simulink model "RL_SAC"  (R2025a)
settings: Solver=FixedStepDiscrete  StartTime=0.0  StopTime=20  FixedStep=1e-2  RelTol=1e-6
undefined symbols (not defined in the file or in its folder): DiscIntNeverNeededParam
libraries: simulink x26, cstblocks x16, slpidlib x2, aerolibutil x2, rllib x1
(part 1 of 2)
settings Model: Creator=Rewse  LastModifiedBy=Rewse
settings SolverCC: ZeroCrossAlgorithm=Adaptive
settings DebuggingCC: IgnoredZcDiagnostic=none

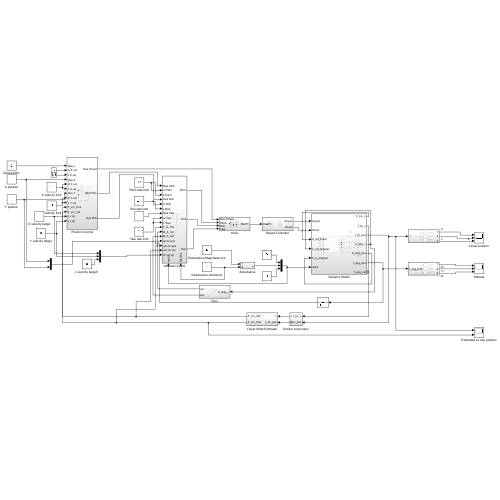
[thumbnail: Simulink's stored preview of the top-level diagram]
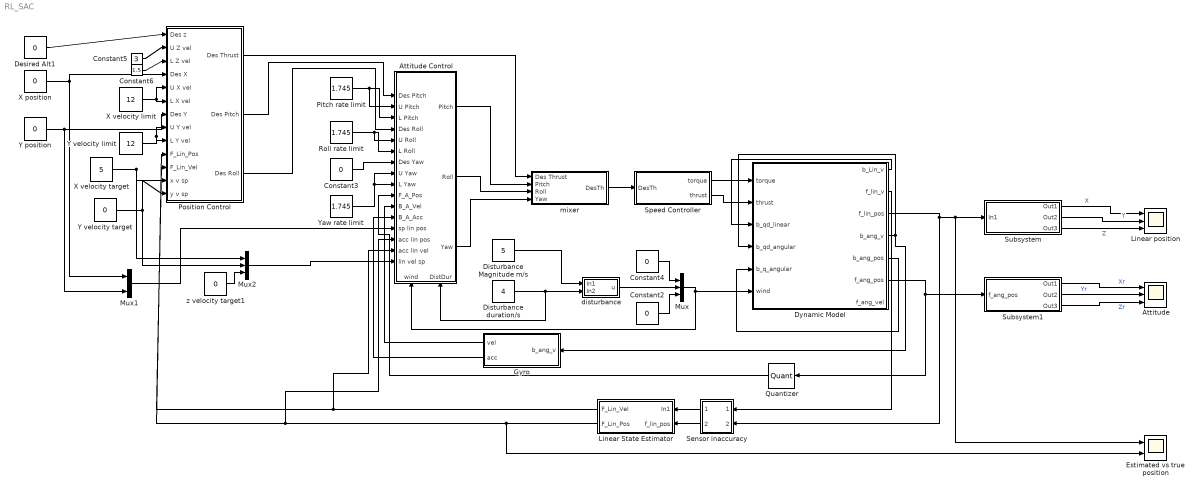
== system RL_SAC ==
  Attitude : Scope  NumInputPorts=3
      settings: ActiveDisplayYMinimum=-0.14361706032504082  ActiveDisplayYMaximum=0.032180546119047609
  Attitude Control : Subsystem
      settings: PortSchema="{\"entries\":[{\"content\":{\"sides\":[{\"content\":{\"connectorIds\":[\"In1\",\"In2\",\"In3\",\"In4\",\"In5\",\"In6\",\"In7\",\"In8\",\"In9\",\"In10\",\"In11\",\"In12\",\"In13\",\"In14\",\"In15\",\"In16\"]},\"type\":\"ConnectorPlacement.EquallySpacedRectSide\",\"uuid\":\"5aea7e22-cf15-44ef-b205-b6ced6f298a4\"},{\"content\":{\"connectorIds\":[\"Out1\",\"Out2\",\"Out3\"],\"side\":\"RIGHT\"},\"type\":\"ConnectorPlacement.EquallySpacedRectSide\",\"uuid\":\"9ef0269e-c37e-412a-be4f-a3e367ef4d40\"},{\"content\":{\"side\":\"TOP\"},\"type\":\"ConnectorPlacement.EquallySpacedRectSide\",\"uuid\":\"5b75e127-dd51-46ce-894a-a13043237b79\"},{\"content\":{\"connectorIds\":[\"In17\",\"In18\"],\"side\":\"BOTTOM\"},\"type\":\"ConnectorPlacement.EquallySpacedRectSide\",\"uuid\":\"a8713bdf-8295-4b8e-972b-b20a63c171f4\"}]},\"type\":\"ConnectorPlacement.EquallySpacedConnector\",\"uuid\":\"ff6dc2c6-b6a3-43bc-805b-8e42f8232d67\"}],\"packageUris\":[\"http://schema.mathworks.com/mf0/Connector/R2020b\"],\"version\":\"1.0\"}"
  Constant2 : Constant  Value=0
  Constant3 : Constant  Value=0
  Constant4 : Constant  Value=0
  Constant5 : Constant  Value=3
  Constant6 : Constant  Value=1.5
  Desired Alt1 : Constant  Value=0
  Disturbance Magnitude m/s : Constant  Value=5
  Disturbance duration/s : Constant  Value=4
  Dynamic Model : Subsystem
  Estimated vs true position : Scope  NumInputPorts=2
      settings: ActiveDisplayYMinimum=-18.877528524364443  ActiveDisplayYMaximum=162.40656098897554  DataLoggingVariableName=ScopeData4
  Gyro : Subsystem
  Linear State Estimator : Subsystem
  Linear position : Scope  NumInputPorts=3
      settings: ActiveDisplayYMinimum=-25.0677489650157  ActiveDisplayYMaximum=225.60952843294078
  Mux : Mux  Inputs=3
  Mux1 : Mux  Inputs=2
  Mux2 : Mux  Inputs=3
  Pitch rate limit : Constant  Value=1.745
  Position Control : Subsystem
  Quantizer : Quantizer  QuantizationInterval=0.01
  Roll rate limit : Constant  Value=1.745
  Sensor inaccuracy : Subsystem
  Speed Controller : Subsystem
  Subsystem : Subsystem
  Subsystem1 : Subsystem
  X position : Constant  Value=0
  X velocity limit : Constant  Value=12
  X velocity target : Constant  Value=5
  Y position : Constant  Value=0
  Y velocity limit : Constant  Value=12
  Y velocity target : Constant  Value=0
  Yaw rate limit : Constant  Value=1.745
  disturbance : Subsystem
  mixer : Subsystem
  z velocity target1 : Constant  Value=0
  wires:
  Subsystem/1(Out1) -> Linear position/1  "X"
  Subsystem/2(Out2) -> Linear position/2  "Y"
  Subsystem/3(Out3) -> Linear position/3  "Z"
  Subsystem1/1(Out1) -> Attitude/1  "Xr"
  Subsystem1/2(Out2) -> Attitude/2  "Yr"
  Subsystem1/3(Out3) -> Attitude/3  "Zr"
  Dynamic Model/5(b_ang_pos) -> Dynamic Model/5(b_q_angular)
  Dynamic Model/1(b_Lin_v) -> Dynamic Model/3(b_qd_linear)
  mixer/1(DesTh) -> Speed Controller/1(DesTh)
  Dynamic Model/4(b_ang_v) -> Gyro/1(b_ang_v), Dynamic Model/4(b_qd_angular)
  Attitude Control/1(Pitch) -> mixer/2(Pitch)
  Attitude Control/2(Roll) -> mixer/3(Roll)
  Pitch rate limit/1 -> Attitude Control/3(L Pitch), Attitude Control/2(U Pitch)
  Roll rate limit/1 -> Attitude Control/6(L Roll), Attitude Control/5(U Roll)
  Yaw rate limit/1 -> Attitude Control/8(U Yaw), Attitude Control/9(L Yaw)
  Constant3/1 -> Attitude Control/7(Des Yaw)
  Speed Controller/2(thrust) -> Dynamic Model/2(thrust)
  Speed Controller/1(torque) -> Dynamic Model/1(torque)
  Constant5/1 -> Position Control/2(U Z vel)
  Desired Alt1/1 -> Position Control/1(Des z)
  X velocity limit/1 -> Position Control/6(L X vel), Position Control/5(U X vel)
  Y velocity limit/1 -> Position Control/9(L Y vel), Position Control/8(U Y vel)
  Position Control/1(Des Thrust) -> mixer/1(Des Thrust)
  Constant6/1 -> Position Control/3(L Z vel)
  Y position/1 -> Mux1/2, Position Control/7(Des Y)
  Attitude Control/3(Yaw) -> mixer/4(Yaw)
  Gyro/1(vel) -> Attitude Control/11(B_A_Vel)
  Gyro/2(acc) -> Attitude Control/12(B_A_Acc)
  Dynamic Model/6(f_ang_pos) -> Quantizer/1, Subsystem1/1(f_ang_pos)
  X position/1 -> Mux1/1, Position Control/4(Des X)
  Constant2/1 -> Mux/3
  Sensor inaccuracy/2(Out2) -> Linear State Estimator/2(f_lin_pos)
  Sensor inaccuracy/1(Out1) -> Linear State Estimator/1(In1)
  Dynamic Model/2(f_lin_v) -> Sensor inaccuracy/1(f_lin_v)
  Dynamic Model/3(f_lin_pos) -> Sensor inaccuracy/2(f_lin_pos), Estimated vs true position/1, Subsystem/1(In1)
  Position Control/3(Des Roll) -> Attitude Control/4(Des Roll)
  Position Control/2(Des Pitch) -> Attitude Control/1(Des Pitch)
  Linear State Estimator/1(F_Lin_Vel) -> Attitude Control/15(acc lin vel), Position Control/11(F_Lin_Vel)
  Linear State Estimator/2(F_Lin_Pos) -> Estimated vs true position/2, Position Control/10(F_Lin_Pos), Attitude Control/14(acc lin pos)
  Mux1/1 -> Attitude Control/13(sp lin pos)
  Mux/1 -> Dynamic Model/6(wind), Attitude Control/17(wind)
  X velocity target/1 -> Mux2/1, Position Control/12(x v sp)
  Y velocity target/1 -> Mux2/2, Position Control/13(y v sp)
  Constant4/1 -> Mux/1
  Mux2/1 -> Attitude Control/16(lin vel sp)
  z velocity target1/1 -> Mux2/3
  Disturbance Magnitude m/s/1 -> disturbance/1(In1)
  disturbance/1(u) -> Mux/2
  Quantizer/1 -> Attitude Control/10(F_A_Pos)
  Disturbance duration/s/1 -> disturbance/2(In2), Attitude Control/18(DistDur)

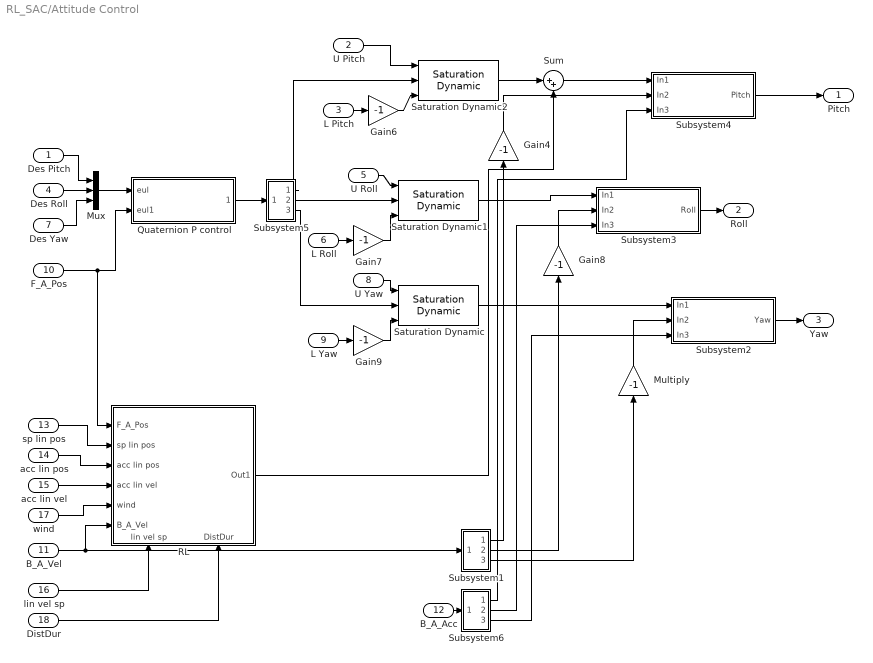
== system RL_SAC/Attitude Control ==
  Des Pitch : Inport
  U Pitch : Inport  Port=2
  L Pitch : Inport  Port=3
  Des Roll : Inport  Port=4
  U Roll : Inport  Port=5
  L Roll : Inport  Port=6
  Des Yaw : Inport  Port=7
  U Yaw : Inport  Port=8
  L Yaw : Inport  Port=9
  F_A_Pos : Inport  Port=10
  B_A_Vel : Inport  Port=11
  B_A_Acc : Inport  Port=12
  sp lin pos : Inport  Port=13
  acc lin pos : Inport  Port=14
  acc lin vel : Inport  Port=15
  lin vel sp : Inport  Port=16
  wind : Inport  Port=17
  DistDur : Inport  Port=18
  Gain{4,6..9} (5 alike) : Gain  Gain=-1
  Multiply : Gain  Gain=-1
  Mux : Mux  Inputs=3
  Quaternion P control : Subsystem
  RL : Subsystem
      settings: PortSchema="{\"entries\":[{\"content\":{\"sides\":[{\"content\":{\"connectorIds\":[\"In1\",\"In2\",\"In3\",\"In4\",\"In5\",\"In6\"]},\"type\":\"ConnectorPlacement.EquallySpacedRectSide\",\"uuid\":\"de9c2034-cd13-466b-8304-909c4731cac8\"},{\"content\":{\"connectorIds\":[\"Out1\"],\"side\":\"RIGHT\"},\"type\":\"ConnectorPlacement.EquallySpacedRectSide\",\"uuid\":\"4bbf1dae-6c36-474f-8444-ba23edf5e83e\"},{\"content\":{\"side\":\"TOP\"},\"type\":\"ConnectorPlacement.EquallySpacedRectSide\",\"uuid\":\"e128e6e1-e112-4b3d-a554-370c1b41a3dc\"},{\"content\":{\"connectorIds\":[\"In7\",\"In8\"],\"side\":\"BOTTOM\"},\"type\":\"ConnectorPlacement.EquallySpacedRectSide\",\"uuid\":\"ffd3f57f-9382-4033-b19c-cb1eae5b476f\"}]},\"type\":\"ConnectorPlacement.EquallySpacedConnector\",\"uuid\":\"d8782a20-2727-49b0-a468-40b427850214\"}],\"packageUris\":[\"http://schema.mathworks.com/mf0/Connector/R2020b\"],\"version\":\"1.0\"}"
  Saturation Dynamic : simulink/Discontinuities/Saturation Dynamic  OutMin=[]  OutMax=[]  OutDataTypeStr=Inherit: Same as second input  OutDataType=fixdt(1, 16)  OutScaling=2^-10  DoSatur=off
  Saturation Dynamic1 : simulink/Discontinuities/Saturation Dynamic  OutMin=[]  OutMax=[]  OutDataTypeStr=Inherit: Same as second input  OutDataType=fixdt(1, 16)  OutScaling=2^-10  DoSatur=off
  Saturation Dynamic2 : simulink/Discontinuities/Saturation Dynamic  OutMin=[]  OutMax=[]  OutDataTypeStr=Inherit: Same as second input  OutDataType=fixdt(1, 16)  OutScaling=2^-10  DoSatur=off
  Subsystem1 : Subsystem
  Subsystem2 : Subsystem
  Subsystem3 : Subsystem
  Subsystem4 : Subsystem
  Subsystem5 : Subsystem
  Subsystem6 : Subsystem
  Sum : Sum  Inputs=|++
  Pitch : Outport
  Roll : Outport  Port=2
  Yaw : Outport  Port=3
  wires:
  Gain9/1 -> Saturation Dynamic/3
  Gain6/1 -> Saturation Dynamic2/3
  Gain7/1 -> Saturation Dynamic1/3
  B_A_Vel/1 -> Subsystem1/1("  "), RL/6(B_A_Vel)
  U Roll/1 -> Saturation Dynamic1/1
  L Pitch/1 -> Gain6/1
  U Pitch/1 -> Saturation Dynamic2/1
  Subsystem1/1(Out1) -> Gain4/1
  Subsystem1/2(Out2) -> Gain8/1
  Subsystem1/3(Out3) -> Multiply/1
  Saturation Dynamic/1 -> Subsystem2/1(In1)
  Gain8/1 -> Subsystem3/2(In2)
  Subsystem2/1(Yaw) -> Yaw/1
  Multiply/1 -> Subsystem2/2(In2)
  Gain4/1 -> Subsystem4/2(In2)
  Subsystem4/1(Pitch) -> Pitch/1
  Saturation Dynamic1/1 -> Subsystem3/1(In1)
  Subsystem3/1(Roll) -> Roll/1
  L Yaw/1 -> Gain9/1
  Des Roll/1 -> Mux/2
  Des Yaw/1 -> Mux/3
  U Yaw/1 -> Saturation Dynamic/1
  Subsystem5/3(Out3) -> Saturation Dynamic/2
  Subsystem5/2(Out2) -> Saturation Dynamic1/2
  Mux/1 -> Quaternion P control/1(eul)
  F_A_Pos/1 -> RL/1(F_A_Pos), Quaternion P control/2(eul1)
  Quaternion P control/1("  ") -> Subsystem5/1("  ")
  L Roll/1 -> Gain7/1
  B_A_Acc/1 -> Subsystem6/1("  ")
  Subsystem6/1(Out1) -> Subsystem4/3(In3)
  Subsystem6/2(Out2) -> Subsystem3/3(In3)
  Subsystem6/3(Out3) -> Subsystem2/3(In3)
  sp lin pos/1 -> RL/2(sp lin pos)
  acc lin pos/1 -> RL/3(acc lin pos)
  acc lin vel/1 -> RL/4(acc lin vel)
  wind/1 -> RL/5(wind)
  lin vel sp/1 -> RL/7(lin vel sp)
  Subsystem5/1(Out1) -> Saturation Dynamic2/2
  Des Pitch/1 -> Mux/1
  Saturation Dynamic2/1 -> Sum/1
  Sum/1 -> Subsystem4/1(In1)
  RL/1(Out1) -> Sum/2
  DistDur/1 -> RL/8(DistDur)

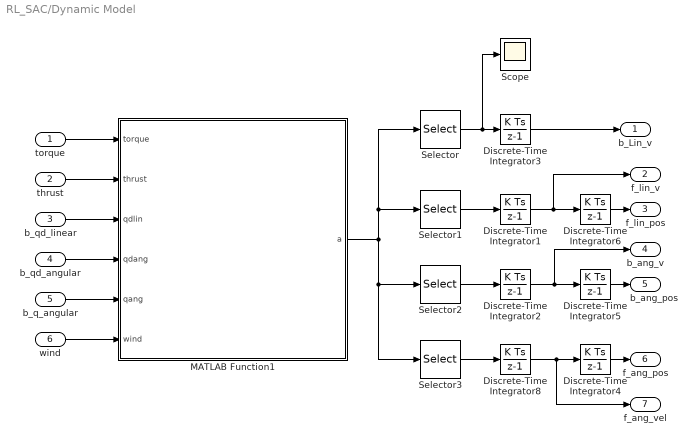
== system RL_SAC/Dynamic Model ==
  torque : Inport
  thrust : Inport  Port=2
  b_qd_linear : Inport  Port=3
  b_qd_angular : Inport  Port=4
  b_q_angular : Inport  Port=5
  wind : Inport  Port=6
  Discrete-Time Integrator1 : DiscreteIntegrator  InitialCondition=[10;0;0]  SampleTime=-1  ICPrevOutput=DiscIntNeverNeededParam  ICPrevScaledInput=DiscIntNeverNeededParam
  Discrete-Time Integrator{2,5..6,8} (4 alike) : DiscreteIntegrator  SampleTime=-1  ICPrevOutput=DiscIntNeverNeededParam  ICPrevScaledInput=DiscIntNeverNeededParam
  Discrete-Time Integrator3 : DiscreteIntegrator  InitialCondition=[0;0;0]  SampleTime=-1  ICPrevOutput=DiscIntNeverNeededParam  ICPrevScaledInput=DiscIntNeverNeededParam
  Discrete-Time Integrator4 : DiscreteIntegrator  InitialCondition=[0;-0.785;0]  SampleTime=-1  ICPrevOutput=DiscIntNeverNeededParam  ICPrevScaledInput=DiscIntNeverNeededParam
  MATLAB Function1 : MATLAB Function  TreatAsAtomicUnit=on
  Scope : Scope
      settings: ActiveDisplayYMinimum=-1  ActiveDisplayYMaximum=1  DataLoggingVariableName=ScopeData3
  Selector : Selector  InputPortWidth=12  IndexOptions=Index vector (dialog)  Indices=[1 2 3]  OutputSizes=1
  Selector1 : Selector  InputPortWidth=12  IndexOptions=Index vector (dialog)  Indices=[4 5 6]  OutputSizes=1
  Selector2 : Selector  InputPortWidth=12  IndexOptions=Index vector (dialog)  Indices=[7 8 9]  OutputSizes=1
  Selector3 : Selector  InputPortWidth=12  IndexOptions=Index vector (dialog)  Indices=[10 11 12]  OutputSizes=1
  b_Lin_v : Outport
  f_lin_v : Outport  Port=2
  f_lin_pos : Outport  Port=3
  b_ang_v : Outport  Port=4
  b_ang_pos : Outport  Port=5
  f_ang_pos : Outport  Port=6
  f_ang_vel : Outport  Port=7
  wires:
  torque/1 -> MATLAB Function1/1(torque)
  thrust/1 -> MATLAB Function1/2(thrust)
  b_qd_linear/1 -> MATLAB Function1/3(qdlin)
  b_qd_angular/1 -> MATLAB Function1/4(qdang)
  b_q_angular/1 -> MATLAB Function1/5(qang)
  wind/1 -> MATLAB Function1/6(wind)
  MATLAB Function1/1(a) -> Selector1/1, Selector/1, Selector3/1, Selector2/1
  Selector/1 -> Scope/1, Discrete-Time Integrator3/1
  Selector1/1 -> Discrete-Time Integrator1/1
  Selector2/1 -> Discrete-Time Integrator2/1
  Selector3/1 -> Discrete-Time Integrator8/1
  Discrete-Time Integrator3/1 -> b_Lin_v/1
  Discrete-Time Integrator2/1 -> b_ang_v/1, Discrete-Time Integrator5/1
  Discrete-Time Integrator1/1 -> Discrete-Time Integrator6/1, f_lin_v/1
  Discrete-Time Integrator8/1 -> f_ang_vel/1, Discrete-Time Integrator4/1
  Discrete-Time Integrator4/1 -> f_ang_pos/1
  Discrete-Time Integrator5/1 -> b_ang_pos/1
  Discrete-Time Integrator6/1 -> f_lin_pos/1

== system RL_SAC/Gyro ==
  b_ang_v : Inport
  Constant1 : Constant  Value=40
  Constant7 : Constant  Value=40
  Discrete Derivative : simulink/Discrete/Discrete Derivative  gainval=1.0  ICPrevScaledInput=0.0  OutMin=[]  OutMax=[]  OutDataType=fixdt(1, 16)  OutScaling=2^-10  DoSatur=off
  Discrete Varying Lowpass : cstblocks/Linear Parameter Varying/Discrete Varying Lowpass  N=2  w0=0  Ts=1e-2
  Discrete Varying Lowpass1 : cstblocks/Linear Parameter Varying/Discrete Varying Lowpass  N=2  w0=0  Ts=1e-2
  Quantizer : Quantizer  QuantizationInterval=0.00026179939
  noise : Subsystem
  vel : Outport
  acc : Outport  Port=2
  wires:
  Constant1/1 -> Discrete Varying Lowpass1/2
  Quantizer/1 -> Discrete Varying Lowpass/1
  Discrete Derivative/1 -> Discrete Varying Lowpass1/1
  Constant7/1 -> Discrete Varying Lowpass/2
  Discrete Varying Lowpass/1 -> vel/1, Discrete Derivative/1
  b_ang_v/1 -> noise/1(In1)
  noise/1(Out1) -> Quantizer/1
  Discrete Varying Lowpass1/1 -> acc/1

== system RL_SAC/Linear State Estimator ==
  In1 : Inport
  f_lin_pos : Inport  Port=2
  Complimentary filter : Subsystem
  Constant7 : Constant  Value=10
  Discrete Varying Lowpass1 : cstblocks/Linear Parameter Varying/Discrete Varying Lowpass  N=2  w0=0  Ts=1e-2
  F_Lin_Vel : Outport
  F_Lin_Pos : Outport  Port=2
  wires:
  In1/1 -> Discrete Varying Lowpass1/1, Complimentary filter/1(In1)
  f_lin_pos/1 -> Complimentary filter/2(f_lin_pos)
  Complimentary filter/1(F_Lin_Pos) -> F_Lin_Pos/1
  Discrete Varying Lowpass1/1 -> F_Lin_Vel/1
  Constant7/1 -> Discrete Varying Lowpass1/2

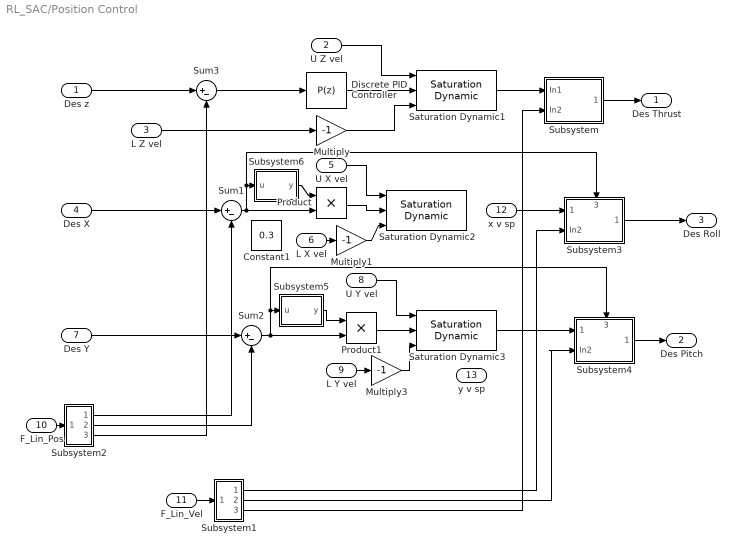
== system RL_SAC/Position Control ==
  Des z : Inport
  U Z vel : Inport  Port=2
  L Z vel : Inport  Port=3
  Des X : Inport  Port=4
  U X vel : Inport  Port=5
  L X vel : Inport  Port=6
  Des Y : Inport  Port=7
  U Y vel : Inport  Port=8
  L Y vel : Inport  Port=9
  F_Lin_Pos : Inport  Port=10
  F_Lin_Vel : Inport  Port=11
  x v sp : Inport  Port=12
  y v sp : Inport  Port=13
  Constant1 : Constant  Value=0.3
  Discrete PID Controller : slpidlib/PID Controller  Controller=P  Form=Parallel  TimeDomain=Discrete-time  UseExternalTs=off  SampleTime=-1  IntegratorMethod=Forward Euler  FilterMethod=Forward Euler  ControllerParametersSource=internal  P=4  I=0.2  UseKiTs=off  D=1  UseExternalDerivativeSource=off  N=100  UseFilter=on  TunerSelectOption=Transfer Function Based (PID Tuner App)  InitialConditionSource=internal  InitialConditionForIntegrator=0  InitialConditionForFilter=0  DifferentiatorICPrevScaledInput=0  ExternalReset=none  TrackingMode=off  Kt=1  LimitOutput=off  SatLimitsSource=internal  UpperSaturationLimit=inf  LowerSaturationLimit=-inf  LinearizeAsGain=off  AntiWindupMode=none  Kb=1  LimitIntegrator=off  UpperIntegratorSaturationLimit=inf  LowerIntegratorSaturationLimit=-inf  POutMin=[]  POutMax=[]  IOutMin=[]  IOutMax=[]  DOutMin=[]  DOutMax=[]  NOutMin=[]  NOutMax=[]  SumOutMin=[]  SumOutMax=[]  SaturationOutMin=[]  SaturationOutMax=[]  PParamMin=[]  PParamMax=[]  IParamMin=[]  IParamMax=[]  DParamMin=[]  DParamMax=[]  NParamMin=[]  NParamMax=[]  KbParamMin=[]  KbParamMax=[]  KtParamMin=[]  KtParamMax=[]  KbOutMin=[]  KbOutMax=[]  KtOutMin=[]  KtOutMax=[]  IntegratorOutMin=[]  IntegratorOutMax=[]  FilterOutMin=[]  FilterOutMax=[]  SumI1OutMin=[]  SumI1OutMax=[]  SumI2OutMin=[]  SumI2OutMax=[]  SumI3OutMin=[]  SumI3OutMax=[]  SumI4OutMin=[]  SumI4OutMax=[]  SumDOutMin=[]  SumDOutMax=[]  DifferentiatorOutMin=[]  DifferentiatorOutMax=[]  FilterDiffOutCoefMin=[]  FilterDiffOutCoefMax=[]  ReciprocalOutMin=[]  ReciprocalOutMax=[]  SumDenOutMin=[]  SumDenOutMax=[]  SumNumOutMin=[]  SumNumOutMax=[]  DivideOutMin=[]  DivideOutMax=[]  UdiffTsProdOutMin=[]  UdiffTsProdOutMax=[]  NTsProdOutMin=[]  NTsProdOutMax=[]  UintegralTsProdOutMin=[]  UintegralTsProdOutMax=[]  UngainTsProdOutMin=[]  UngainTsProdOutMax=[]  ClampingZeroOutDataTypeStr=Inherit: Inherit via back propagation  ClampingZeroOutMin=[]  ClampingZeroOutMax=[]  FilterDenConstantOutDataTypeStr=Inherit: Inherit via back propagation  FilterDenConstantOutMin=[]  FilterDenConstantOutMax=[]  PCopyOutDataTypeStr=Inherit: Inherit via back propagation  PCopyOutMin=[]  PCopyOutMax=[]  NCopyOutDataTypeStr=Inherit: Inherit via back propagation  NCopyOutMin=[]  NCopyOutMax=[]  IntegratorContinuousStateAttributes=''  IntegratorStateMustResolveToSignalObject=off  IntegratorRTWStateStorageClass=Auto  FilterContinuousStateAttributes=''  FilterStateMustResolveToSignalObject=off  FilterRTWStateStorageClass=Auto  ParallelPVariant=InternalParameters  IdealPVariant=Disabled  IVariant=Disabled  DVariant=Disabled  IntegratorVariant=Disabled  SatVariant=Disabled  AWVariant=Disabled  PCopyVariant=Disabled  TRVariant=Disabled  FdbkBlocksVariant=Forward  IdealPFdbkVariant=Disabled  SatFdbkVariant=Disabled  DerivativeFilterVariant=Disabled  NVariant=Disabled  NCopyVariant=Disabled_SignalSpec  FilterICVariant=Disabled  IntegratorICVariant=Disabled  ExternalResetVariant=Disabled  TRSumVariant=Passthrough  SumFdbkVariant=Disabled  SumVariant=Passthrough_P  TsampFilterVariant=InternalTs  TsampNgainVariant=Passthrough  TsampIntegralVariant=Disabled_SignalSpec  ExternalSaturationOutDataTypeStr=Inherit: Same as second input  DerivativeSourceVariant=Disabled  PreIntVariant=InternalPreInt
      settings: LibrarySourceBlock=simulink/Discrete/Discrete PID Controller
  Multiply : Gain  Gain=-1
  Multiply1 : Gain  Gain=-1
  Multiply3 : Gain  Gain=-1
  Product : Product
  Product1 : Product
  Saturation Dynamic1 : simulink/Discontinuities/Saturation Dynamic  OutMin=[]  OutMax=[]  OutDataTypeStr=Inherit: Same as second input  OutDataType=fixdt(1, 16)  OutScaling=2^-10  DoSatur=off
  Saturation Dynamic2 : simulink/Discontinuities/Saturation Dynamic  OutMin=[]  OutMax=[]  OutDataTypeStr=Inherit: Same as second input  OutDataType=fixdt(1, 16)  OutScaling=2^-10  DoSatur=off
  Saturation Dynamic3 : simulink/Discontinuities/Saturation Dynamic  OutMin=[]  OutMax=[]  OutDataTypeStr=Inherit: Same as second input  OutDataType=fixdt(1, 16)  OutScaling=2^-10  DoSatur=off
  Subsystem : Subsystem
  Subsystem1 : Subsystem
  Subsystem2 : Subsystem
  Subsystem3 : Subsystem
      settings: PortSchema="{\"entries\":[{\"content\":{\"sides\":[{\"content\":{\"connectorIds\":[\"In1\",\"In2\"]},\"type\":\"ConnectorPlacement.EquallySpacedRectSide\",\"uuid\":\"8f94e582-882b-486f-b435-c6f08064346b\"},{\"content\":{\"connectorIds\":[\"Out1\"],\"side\":\"RIGHT\"},\"type\":\"ConnectorPlacement.EquallySpacedRectSide\",\"uuid\":\"472883df-7159-496e-9a5d-2a26c086a4a5\"},{\"content\":{\"connectorIds\":[\"In3\"],\"side\":\"TOP\"},\"type\":\"ConnectorPlacement.EquallySpacedRectSide\",\"uuid\":\"9ed532c8-9328-48c4-bd89-739726c76bc0\"}]},\"type\":\"ConnectorPlacement.EquallySpacedConnector\",\"uuid\":\"e990e484-f5ed-4898-afa7-038328da9bdf\"}],\"packageUris\":[\"http://schema.mathworks.com/mf0/Connector/R2020b\"],\"version\":\"1.0\"}"
  Subsystem4 : Subsystem
      settings: PortSchema="{\"entries\":[{\"content\":{\"sides\":[{\"content\":{\"connectorIds\":[\"In1\",\"In2\"]},\"type\":\"ConnectorPlacement.EquallySpacedRectSide\",\"uuid\":\"8f94e582-882b-486f-b435-c6f08064346b\"},{\"content\":{\"connectorIds\":[\"Out1\"],\"side\":\"RIGHT\"},\"type\":\"ConnectorPlacement.EquallySpacedRectSide\",\"uuid\":\"472883df-7159-496e-9a5d-2a26c086a4a5\"},{\"content\":{\"connectorIds\":[\"In3\"],\"side\":\"TOP\"},\"type\":\"ConnectorPlacement.EquallySpacedRectSide\",\"uuid\":\"9ed532c8-9328-48c4-bd89-739726c76bc0\"}]},\"type\":\"ConnectorPlacement.EquallySpacedConnector\",\"uuid\":\"e990e484-f5ed-4898-afa7-038328da9bdf\"}],\"packageUris\":[\"http://schema.mathworks.com/mf0/Connector/R2020b\"],\"version\":\"1.0\"}"
  Subsystem5 : Subsystem
  Subsystem6 : Subsystem
  Sum1 : Sum  Inputs=|+-
  Sum2 : Sum  Inputs=|+-
  Sum3 : Sum  Inputs=|+-
  Des Thrust : Outport
  Des Pitch : Outport  Port=2
  Des Roll : Outport  Port=3
  wires:
  Sum3/1 -> Discrete PID Controller/1
  Multiply/1 -> Saturation Dynamic1/3
  Des z/1 -> Sum3/1
  Discrete PID Controller/1 -> Saturation Dynamic1/2
  L Z vel/1 -> Multiply/1
  U Z vel/1 -> Saturation Dynamic1/1
  Saturation Dynamic1/1 -> Subsystem/1(In1)
  F_Lin_Vel/1 -> Subsystem1/1("  ")
  F_Lin_Pos/1 -> Subsystem2/1("  ")
  Subsystem2/3(Out3) -> Sum3/2
  Subsystem1/3(Out3) -> Subsystem/2(In2)
  Subsystem/1(Des Thrust) -> Des Thrust/1
  Des X/1 -> Sum1/1
  Sum1/1 -> Subsystem3/3(3), Subsystem6/1(u), Product/2
  Product/1 -> Saturation Dynamic2/2
  U X vel/1 -> Saturation Dynamic2/1
  Multiply1/1 -> Saturation Dynamic2/3
  L X vel/1 -> Multiply1/1
  L Y vel/1 -> Multiply3/1
  Multiply3/1 -> Saturation Dynamic3/3
  Sum2/1 -> Subsystem5/1(u), Subsystem4/3(3), Product1/2
  Product1/1 -> Saturation Dynamic3/2
  Subsystem4/1(Des Pitch) -> Des Pitch/1
  Des Y/1 -> Sum2/1
  U Y vel/1 -> Saturation Dynamic3/1
  Subsystem1/1(Out1) -> Subsystem3/2(In2)
  Subsystem2/2(Out1) -> Sum2/2
  Subsystem2/1(Out2) -> Sum1/2
  Subsystem3/1(Des Roll) -> Des Roll/1
  Subsystem6/1(y) -> Product/1
  Subsystem5/1(y) -> Product1/1
  Subsystem1/2(Out2) -> Subsystem4/2(In2)
  Saturation Dynamic3/1 -> Subsystem4/1(y v sp)
  x v sp/1 -> Subsystem3/1(x v sp)

== system RL_SAC/Sensor inaccuracy ==
  f_lin_v : Inport
  f_lin_pos : Inport  Port=2
  Quantizer : Quantizer  QuantizationInterval=0.01
  Quantizer1 : Quantizer  QuantizationInterval=1
  Out1 : Outport
  Out2 : Outport  Port=2
  wires:
  f_lin_v/1 -> Quantizer/1
  f_lin_pos/1 -> Quantizer1/1
  Quantizer1/1 -> Out2/1
  Quantizer/1 -> Out1/1

== system RL_SAC/Speed Controller ==
  DesTh : Inport
  Rotor 1 : Subsystem
  Rotor 2 : Subsystem
  Rotor 3 : Subsystem
  Rotor 4 : Subsystem
  Saturation{,1..3} (4 alike) : Saturate  UpperLimit=8.96325  LowerLimit=0
  Selector2 : Selector  InputPortWidth=4  IndexOptions=Index vector (dialog)  Indices=[1]  OutputSizes=1
  Selector3 : Selector  InputPortWidth=4  IndexOptions=Index vector (dialog)  Indices=[2]  OutputSizes=1
  Selector4 : Selector  InputPortWidth=4  IndexOptions=Index vector (dialog)  Indices=[3]  OutputSizes=1
  Selector5 : Selector  InputPortWidth=4  IndexOptions=Index vector (dialog)  Indices=[4]  OutputSizes=1
  Subsystem : Subsystem
  torque : Outport
  thrust : Outport  Port=2
  wires:
  Selector5/1 -> Saturation3/1
  Selector2/1 -> Saturation/1
  Selector3/1 -> Saturation1/1
  Selector4/1 -> Saturation2/1
  Saturation/1 -> Rotor 1/1(Desired_Thrust)
  Saturation1/1 -> Rotor 2/1(Desired_Thrust)
  Saturation2/1 -> Rotor 3/1(Desired_Thrust)
  Saturation3/1 -> Rotor 4/1(Desired_Thrust)
  Rotor 2/2(Rotor Thrust) -> Subsystem/4(In4)
  Rotor 3/2(Rotor Thrust) -> Subsystem/6(In6)
  Rotor 4/2(Rotor Thrust) -> Subsystem/8(In8)
  Rotor 1/2(Rotor Thrust) -> Subsystem/2(Rotor Thrust)
  Rotor 1/1(Rotor Torque) -> Subsystem/1(Rotor Torque)
  Rotor 2/1(Rotor Torque) -> Subsystem/3(In3)
  Rotor 3/1(Rotor Torque) -> Subsystem/5(In5)
  Rotor 4/1(Rotor Torque) -> Subsystem/7(In7)
  Subsystem/1(Out1) -> torque/1
  DesTh/1 -> Selector2/1, Selector3/1, Selector5/1, Selector4/1
  Subsystem/2(thrust) -> thrust/1

== system RL_SAC/Subsystem ==
  In1 : Inport
  Selector1 : Selector  InputPortWidth=3  IndexOptions=Index vector (dialog)  Indices=[2]  OutputSizes=1
  Selector10 : Selector  InputPortWidth=3  IndexOptions=Index vector (dialog)  Indices=[1]  OutputSizes=1
  Selector2 : Selector  InputPortWidth=3  IndexOptions=Index vector (dialog)  Indices=[3]  OutputSizes=1
  Out1 : Outport
  Out2 : Outport  Port=2
  Out3 : Outport  Port=3
  wires:
  Selector10/1 -> Out1/1  "Xpos"
  Selector1/1 -> Out2/1  "Ypos"
  In1/1 -> Selector2/1, Selector10/1, Selector1/1
  Selector2/1 -> Out3/1  "Zpos"

== system RL_SAC/Subsystem1 ==
  f_ang_pos : Inport
  Selector1 : Selector  InputPortWidth=3  IndexOptions=Index vector (dialog)  Indices=[2]  OutputSizes=1
  Selector10 : Selector  InputPortWidth=3  IndexOptions=Index vector (dialog)  Indices=[1]  OutputSizes=1
  Selector2 : Selector  InputPortWidth=3  IndexOptions=Index vector (dialog)  Indices=[3]  OutputSizes=1
  Out1 : Outport
  Out2 : Outport  Port=2
  Out3 : Outport  Port=3
  wires:
  Selector10/1 -> Out1/1  "Xpos"
  Selector1/1 -> Out2/1  "Ypos"
  f_ang_pos/1 -> Selector2/1, Selector10/1, Selector1/1
  Selector2/1 -> Out3/1  "Zpos"

== system RL_SAC/disturbance ==
  In1 : Inport
  In2 : Inport  Port=2
  Add : Sum
  Add1 : Sum
  Constant : Constant  Value=2
  Delay : Delay  DelayLength=200
  Gain : Gain  Gain=-1
  Variable Time Delay : VariableTransportDelay  MaximumDelay=14  MaximumPoints=2048
  u : Outport
  wires:
  Gain/1 -> Variable Time Delay/1
  Delay/1 -> Add/1
  Variable Time Delay/1 -> Add/2
  In1/1 -> Delay/1, Gain/1
  In2/1 -> Add1/1
  Constant/1 -> Add1/2
  Add1/1 -> Variable Time Delay/2
  Add/1 -> u/1

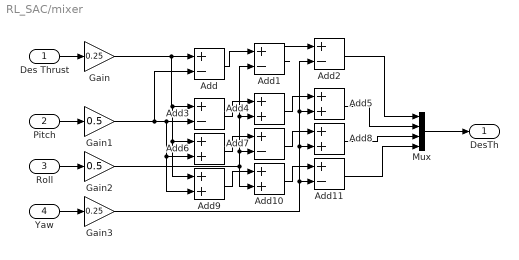
== system RL_SAC/mixer ==
  Des Thrust : Inport
  Pitch : Inport  Port=2
  Roll : Inport  Port=3
  Yaw : Inport  Port=4
  Add{,1..3,7,11} (6 alike) : Sum  Inputs=+-
  Add{4..6,8..10} (6 alike) : Sum
  Gain : Gain  Gain=0.25
  Gain1 : Gain  Gain=0.5
  Gain2 : Gain  Gain=0.5
  Gain3 : Gain  Gain=0.25
  Mux : Mux
  DesTh : Outport
  wires:
  Des Thrust/1 -> Gain/1
  Gain/1 -> Add9/1, Add6/1, Add3/1, Add/1
  Gain1/1 -> Add9/2, Add6/2, Add3/2, Add/2
  Add/1 -> Add1/1
  Gain2/1 -> Add10/2, Add7/2, Add1/2, Add4/2
  Roll/1 -> Gain2/1
  Yaw/1 -> Gain3/1
  Add1/1 -> Add2/1
  Gain3/1 -> Add11/2, Add5/2, Add2/2, Add8/2
  Add2/1 -> Mux/1
  Add3/1 -> Add4/1
  Add4/1 -> Add5/1
  Add5/1 -> Mux/2
  Mux/1 -> DesTh/1
  Add6/1 -> Add7/1
  Add7/1 -> Add8/1
  Add8/1 -> Mux/3
  Add9/1 -> Add10/1
  Add10/1 -> Add11/1
  Add11/1 -> Mux/4
  Pitch/1 -> Gain1/1

== system RL_SAC/Attitude Control/Quaternion P control ==
  eul : Inport
  eul1 : Inport  Port=2
  Discrete PID Controller1 : slpidlib/PID Controller  Controller=P  Form=Parallel  TimeDomain=Discrete-time  UseExternalTs=off  SampleTime=-1  IntegratorMethod=Forward Euler  FilterMethod=Forward Euler  ControllerParametersSource=internal  P=2  I=1  UseKiTs=off  D=0  UseExternalDerivativeSource=off  N=100  UseFilter=on  TunerSelectOption=Transfer Function Based (PID Tuner App)  InitialConditionSource=internal  InitialConditionForIntegrator=0  InitialConditionForFilter=0  DifferentiatorICPrevScaledInput=0  ExternalReset=none  TrackingMode=off  Kt=1  LimitOutput=off  SatLimitsSource=internal  UpperSaturationLimit=inf  LowerSaturationLimit=-inf  LinearizeAsGain=off  AntiWindupMode=none  Kb=1  LimitIntegrator=off  UpperIntegratorSaturationLimit=inf  LowerIntegratorSaturationLimit=-inf  POutMin=[]  POutMax=[]  IOutMin=[]  IOutMax=[]  DOutMin=[]  DOutMax=[]  NOutMin=[]  NOutMax=[]  SumOutMin=[]  SumOutMax=[]  SaturationOutMin=[]  SaturationOutMax=[]  PParamMin=[]  PParamMax=[]  IParamMin=[]  IParamMax=[]  DParamMin=[]  DParamMax=[]  NParamMin=[]  NParamMax=[]  KbParamMin=[]  KbParamMax=[]  KtParamMin=[]  KtParamMax=[]  KbOutMin=[]  KbOutMax=[]  KtOutMin=[]  KtOutMax=[]  IntegratorOutMin=[]  IntegratorOutMax=[]  FilterOutMin=[]  FilterOutMax=[]  SumI1OutMin=[]  SumI1OutMax=[]  SumI2OutMin=[]  SumI2OutMax=[]  SumI3OutMin=[]  SumI3OutMax=[]  SumI4OutMin=[]  SumI4OutMax=[]  SumDOutMin=[]  SumDOutMax=[]  DifferentiatorOutMin=[]  DifferentiatorOutMax=[]  FilterDiffOutCoefMin=[]  FilterDiffOutCoefMax=[]  ReciprocalOutMin=[]  ReciprocalOutMax=[]  SumDenOutMin=[]  SumDenOutMax=[]  SumNumOutMin=[]  SumNumOutMax=[]  DivideOutMin=[]  DivideOutMax=[]  UdiffTsProdOutMin=[]  UdiffTsProdOutMax=[]  NTsProdOutMin=[]  NTsProdOutMax=[]  UintegralTsProdOutMin=[]  UintegralTsProdOutMax=[]  UngainTsProdOutMin=[]  UngainTsProdOutMax=[]  ClampingZeroOutDataTypeStr=Inherit: Inherit via back propagation  ClampingZeroOutMin=[]  ClampingZeroOutMax=[]  FilterDenConstantOutDataTypeStr=Inherit: Inherit via back propagation  FilterDenConstantOutMin=[]  FilterDenConstantOutMax=[]  PCopyOutDataTypeStr=Inherit: Inherit via back propagation  PCopyOutMin=[]  PCopyOutMax=[]  NCopyOutDataTypeStr=Inherit: Inherit via back propagation  NCopyOutMin=[]  NCopyOutMax=[]  IntegratorContinuousStateAttributes=''  IntegratorStateMustResolveToSignalObject=off  IntegratorRTWStateStorageClass=Auto  FilterContinuousStateAttributes=''  FilterStateMustResolveToSignalObject=off  FilterRTWStateStorageClass=Auto  ParallelPVariant=InternalParameters  IdealPVariant=Disabled  IVariant=Disabled  DVariant=Disabled  IntegratorVariant=Disabled  SatVariant=Disabled  AWVariant=Disabled  PCopyVariant=Disabled  TRVariant=Disabled  FdbkBlocksVariant=Forward  IdealPFdbkVariant=Disabled  SatFdbkVariant=Disabled  DerivativeFilterVariant=Disabled  NVariant=Disabled  NCopyVariant=Disabled_SignalSpec  FilterICVariant=Disabled  IntegratorICVariant=Disabled  ExternalResetVariant=Disabled  TRSumVariant=Passthrough  SumFdbkVariant=Disabled  SumVariant=Passthrough_P  TsampFilterVariant=InternalTs  TsampNgainVariant=Passthrough  TsampIntegralVariant=Disabled_SignalSpec  ExternalSaturationOutDataTypeStr=Inherit: Same as second input  DerivativeSourceVariant=Disabled  PreIntVariant=InternalPreInt
      settings: LibrarySourceBlock=simulink/Discrete/Discrete PID Controller
  Gain2 : Gain  Gain=-1
  MATLAB Function : MATLAB Function  TreatAsAtomicUnit=on
  MATLAB Function1 : MATLAB Function  TreatAsAtomicUnit=on
  Product : Product
  Quaternion Inverse : aerolibutil/Quaternion Inverse
  Quaternion Multiplication : aerolibutil/Quaternion Multiplication
  Selector : Selector  InputPortWidth=4  IndexOptions=Index vector (dialog)  Indices=[1]  OutputSizes=1
  Selector1 : Selector  InputPortWidth=4  IndexOptions=Index vector (dialog)  Indices=[2 3 4]  OutputSizes=1
  Sign : Signum
  "  " : Outport
  wires:
  Quaternion Inverse/1 -> Quaternion Multiplication/2
  Selector1/1 -> Product/2
  Product/1 -> Discrete PID Controller1/1
  MATLAB Function/1(quat) -> Quaternion Multiplication/1
  MATLAB Function1/1(quat) -> Quaternion Inverse/1
  Quaternion Multiplication/1 -> Selector1/1, Selector/1
  Selector/1 -> Sign/1
  Discrete PID Controller1/1 -> Gain2/1
  Sign/1 -> Product/1
  Gain2/1 -> "  "/1
  eul/1 -> MATLAB Function/1(eul)
  eul1/1 -> MATLAB Function1/1(eul)

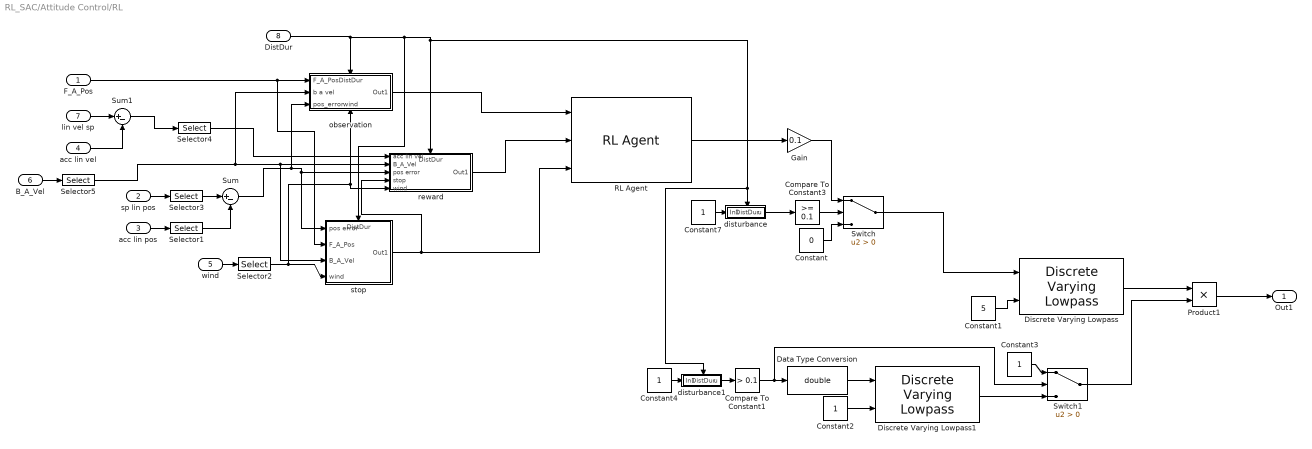
== system RL_SAC/Attitude Control/RL ==
  F_A_Pos : Inport
  sp lin pos : Inport  Port=2
  acc lin pos : Inport  Port=3
  acc lin vel : Inport  Port=4
  wind : Inport  Port=5
  B_A_Vel : Inport  Port=6
  lin vel sp : Inport  Port=7
  DistDur : Inport  Port=8
  Compare To Constant1 : simulink/Logic and Bit Operations/Compare To Constant  relop=>  const=0.1  OutDataTypeStr=boolean
  Compare To Constant3 : simulink/Logic and Bit Operations/Compare To Constant  relop=>=  const=0.1  OutDataTypeStr=boolean
  Constant : Constant  Value=0
  Constant1 : Constant  Value=5
  Constant{2..4,7} (4 alike) : Constant
  Data Type Conversion : DataTypeConversion  OutDataTypeStr=double  SaturateOnIntegerOverflow=off  RndMeth=Floor
  Discrete Varying Lowpass : cstblocks/Linear Parameter Varying/Discrete Varying Lowpass  N=1  w0=0  Ts=1e-2
  Discrete Varying Lowpass1 : cstblocks/Linear Parameter Varying/Discrete Varying Lowpass  N=1  w0=0  Ts=1e-2
  Gain : Gain  Gain=0.1
  Product1 : Product
  RL Agent : rllib/RL Agent  Agent=RLtestSAC3Agent  ExternalActionAsInput=off  ProvideLastAction=off  ProvideCumRwd=off  TreatAsDirectFeedthrough=on  UseStrictObservationDataTypes=off
  Selector1 : Selector  InputPortWidth=3  IndexOptions=Index vector (dialog)  Indices=[2]  OutputSizes=1
  Selector2 : Selector  InputPortWidth=3  IndexOptions=Index vector (dialog)  Indices=[2]  OutputSizes=1
  Selector3 : Selector  InputPortWidth=2  IndexOptions=Index vector (dialog)  Indices=[2]  OutputSizes=1
  Selector4 : Selector  InputPortWidth=3  IndexOptions=Index vector (dialog)  Indices=[2]  OutputSizes=1
  Selector5 : Selector  InputPortWidth=3  IndexOptions=Index vector (dialog)  Indices=[1]  OutputSizes=1
  Sum : Sum  Inputs=|+-
  Sum1 : Sum  Inputs=|+-
  Switch : Switch  Criteria=u2 > Threshold  SaturateOnIntegerOverflow=off  InputSameDT=off
  Switch1 : Switch  Criteria=u2 > Threshold  SaturateOnIntegerOverflow=off  InputSameDT=off
  disturbance : Subsystem
      settings: PortSchema="{\"entries\":[{\"content\":{\"sides\":[{\"content\":{\"connectorIds\":[\"In1\"]},\"type\":\"ConnectorPlacement.EquallySpacedRectSide\",\"uuid\":\"1ea45d97-72cc-4587-9cbf-0adeb2cc8bb7\"},{\"content\":{\"connectorIds\":[\"Out1\"],\"side\":\"RIGHT\"},\"type\":\"ConnectorPlacement.EquallySpacedRectSide\",\"uuid\":\"61165e1b-28cc-48e7-99ef-5ed7ad2a03a2\"},{\"content\":{\"connectorIds\":[\"In2\"],\"side\":\"TOP\"},\"type\":\"ConnectorPlacement.EquallySpacedRectSide\",\"uuid\":\"1ee858fb-66c9-4560-b1d5-e0dc7ce4c9ca\"}]},\"type\":\"ConnectorPlacement.EquallySpacedConnector\",\"uuid\":\"317ef023-ce87-4b82-add9-53b7146a0621\"}],\"packageUris\":[\"http://schema.mathworks.com/mf0/Connector/R2020b\"],\"version\":\"1.0\"}"
  disturbance1 : Subsystem
      settings: PortSchema="{\"entries\":[{\"content\":{\"sides\":[{\"content\":{\"connectorIds\":[\"In1\"]},\"type\":\"ConnectorPlacement.EquallySpacedRectSide\",\"uuid\":\"1ea45d97-72cc-4587-9cbf-0adeb2cc8bb7\"},{\"content\":{\"connectorIds\":[\"Out1\"],\"side\":\"RIGHT\"},\"type\":\"ConnectorPlacement.EquallySpacedRectSide\",\"uuid\":\"61165e1b-28cc-48e7-99ef-5ed7ad2a03a2\"},{\"content\":{\"connectorIds\":[\"In2\"],\"side\":\"TOP\"},\"type\":\"ConnectorPlacement.EquallySpacedRectSide\",\"uuid\":\"1ee858fb-66c9-4560-b1d5-e0dc7ce4c9ca\"}]},\"type\":\"ConnectorPlacement.EquallySpacedConnector\",\"uuid\":\"317ef023-ce87-4b82-add9-53b7146a0621\"}],\"packageUris\":[\"http://schema.mathworks.com/mf0/Connector/R2020b\"],\"version\":\"1.0\"}"
  observation : Subsystem
      settings: PortSchema="{\"entries\":[{\"content\":{\"sides\":[{\"content\":{\"connectorIds\":[\"In1\",\"In2\",\"In3\"]},\"type\":\"ConnectorPlacement.EquallySpacedRectSide\",\"uuid\":\"04f4fe8e-cc6a-4899-a573-8310f200eab6\"},{\"content\":{\"connectorIds\":[\"Out1\"],\"side\":\"RIGHT\"},\"type\":\"ConnectorPlacement.EquallySpacedRectSide\",\"uuid\":\"7d5f31e9-470a-4f58-a705-985aad8c5cc4\"},{\"content\":{\"connectorIds\":[\"In4\"],\"side\":\"TOP\"},\"type\":\"ConnectorPlacement.EquallySpacedRectSide\",\"uuid\":\"11bacbbd-f2b2-4f6c-ae63-90af1039c588\"},{\"content\":{\"connectorIds\":[\"In5\"],\"side\":\"BOTTOM\"},\"type\":\"ConnectorPlacement.EquallySpacedRectSide\",\"uuid\":\"04ec80cb-ae71-47bf-b4e8-187bd859dc0f\"}]},\"type\":\"ConnectorPlacement.EquallySpacedConnector\",\"uuid\":\"9d16dc32-b04a-4dda-aedd-f623cc4c13a8\"}],\"packageUris\":[\"http://schema.mathworks.com/mf0/Connector/R2020b\"],\"version\":\"1.0\"}"
  reward : Subsystem
      settings: PortSchema="{\"entries\":[{\"content\":{\"sides\":[{\"content\":{\"connectorIds\":[\"In1\",\"In2\",\"In3\",\"In4\",\"In5\"]},\"type\":\"ConnectorPlacement.EquallySpacedRectSide\",\"uuid\":\"207526bb-0c8c-497b-bd39-35e0b654f646\"},{\"content\":{\"connectorIds\":[\"Out1\"],\"side\":\"RIGHT\"},\"type\":\"ConnectorPlacement.EquallySpacedRectSide\",\"uuid\":\"a20dfc24-a6e6-4de4-8fac-01421ddc57eb\"},{\"content\":{\"connectorIds\":[\"In6\"],\"side\":\"TOP\"},\"type\":\"ConnectorPlacement.EquallySpacedRectSide\",\"uuid\":\"468e59d5-bbba-48da-b4a6-061d1b240caa\"}]},\"type\":\"ConnectorPlacement.EquallySpacedConnector\",\"uuid\":\"e0236d90-5ee2-4dd0-800e-5a88a8c48159\"}],\"packageUris\":[\"http://schema.mathworks.com/mf0/Connector/R2020b\"],\"version\":\"1.0\"}"
  stop : Subsystem
      settings: PortSchema="{\"entries\":[{\"content\":{\"sides\":[{\"content\":{\"connectorIds\":[\"In1\",\"In2\",\"In3\",\"In4\"]},\"type\":\"ConnectorPlacement.EquallySpacedRectSide\",\"uuid\":\"53290b51-ad63-4d5c-91e6-806ac2060307\"},{\"content\":{\"connectorIds\":[\"Out1\"],\"side\":\"RIGHT\"},\"type\":\"ConnectorPlacement.EquallySpacedRectSide\",\"uuid\":\"b73ee30b-5064-46e0-8317-9085d0ab1cbb\"},{\"content\":{\"connectorIds\":[\"In5\"],\"side\":\"TOP\"},\"type\":\"ConnectorPlacement.EquallySpacedRectSide\",\"uuid\":\"6a6076eb-0597-42ed-9d0b-2932dd8cc85f\"}]},\"type\":\"ConnectorPlacement.EquallySpacedConnector\",\"uuid\":\"4adc0e61-5e79-4118-a24f-94c15939f400\"}],\"packageUris\":[\"http://schema.mathworks.com/mf0/Connector/R2020b\"],\"version\":\"1.0\"}"
  Out1 : Outport
  wires:
  wind/1 -> Selector2/1
  Selector2/1 -> observation/5(wind), reward/5(wind), stop/4(wind)
  B_A_Vel/1 -> Selector5/1
  stop/1(Out1) -> RL Agent/3, reward/4(stop)
  Selector5/1 -> stop/3(B_A_Vel), reward/2(B_A_Vel), observation/2(b a vel)
  Selector4/1 -> reward/1(acc lin vel)
  Compare To Constant3/1 -> Switch/2
  Constant/1 -> Switch/3
  observation/1(Out1) -> RL Agent/1
  lin vel sp/1 -> Sum1/1
  Sum1/1 -> Selector4/1
  F_A_Pos/1 -> stop/2(F_A_Pos), observation/1(F_A_Pos)
  acc lin vel/1 -> Sum1/2
  acc lin pos/1 -> Selector1/1
  sp lin pos/1 -> Selector3/1
  Selector3/1 -> Sum/1
  Selector1/1 -> Sum/2
  Sum/1 -> reward/3(pos error), stop/1(pos error), observation/3(pos_error)
  reward/1(Out1) -> RL Agent/2
  Constant1/1 -> Discrete Varying Lowpass/2
  Constant2/1 -> Discrete Varying Lowpass1/2
  Compare To Constant1/1 -> Switch1/2, Data Type Conversion/1
  Data Type Conversion/1 -> Discrete Varying Lowpass1/1
  Constant3/1 -> Switch1/1
  disturbance/1(u) -> Compare To Constant3/1
  Constant7/1 -> disturbance/1(In1)
  Discrete Varying Lowpass1/1 -> Switch1/3
  Switch1/1 -> Product1/2
  Constant4/1 -> disturbance1/1(In1)
  disturbance1/1(u) -> Compare To Constant1/1
  Gain/1 -> Switch/1
  Switch/1 -> Discrete Varying Lowpass/1
  Discrete Varying Lowpass/1 -> Product1/1
  DistDur/1 -> stop/5(DistDur), disturbance1/2(DistDur), disturbance/2(DistDur), reward/6(DistDur), observation/4(DistDur)
  RL Agent/1 -> Gain/1
  Product1/1 -> Out1/1

== system RL_SAC/Attitude Control/Subsystem1 ==
  "  " : Inport
  Selector : Selector  InputPortWidth=3  IndexOptions=Index vector (dialog)  Indices=[1]  OutputSizes=1
  Selector1 : Selector  InputPortWidth=3  IndexOptions=Index vector (dialog)  Indices=[2]  OutputSizes=1
  Selector2 : Selector  InputPortWidth=3  IndexOptions=Index vector (dialog)  Indices=[3]  OutputSizes=1
  Out1 : Outport
  Out2 : Outport  Port=2
  Out3 : Outport  Port=3
  wires:
  Selector2/1 -> Out3/1
  Selector1/1 -> Out2/1
  Selector/1 -> Out1/1
  "  "/1 -> Selector2/1, Selector/1, Selector1/1

== system RL_SAC/Attitude Control/Subsystem2 ==
  In1 : Inport
  In2 : Inport  Port=2
  In3 : Inport  Port=3
  Add : Sum  Inputs=++-
  Constant : Constant  Value=5
  Discrete Varying Lowpass : cstblocks/Linear Parameter Varying/Discrete Varying Lowpass  N=1  w0=0  Ts=1e-2
  Discrete-Time Integrator : DiscreteIntegrator  SampleTime=-1  ICPrevOutput=DiscIntNeverNeededParam  ICPrevScaledInput=DiscIntNeverNeededParam
  Multiply1 : Gain  Gain=5
  Multiply2 : Gain  Gain=0.1
  Multiply3 : Gain  Gain=0
  Multiply4 : Gain  Gain=0.5
  Saturation2 : Saturate  UpperLimit=20  LowerLimit=-20
  Sum3 : Sum  Inputs=|+-
  Yaw : Outport
  wires:
  In1/1 -> Sum3/1
  Sum3/1 -> Multiply1/1
  In2/1 -> Sum3/2
  Discrete-Time Integrator/1 -> Multiply3/1
  Multiply3/1 -> Add/2
  Discrete Varying Lowpass/1 -> Multiply4/1
  Multiply1/1 -> Add/1, Discrete-Time Integrator/1
  Multiply4/1 -> Add/3
  Add/1 -> Saturation2/1
  Multiply2/1 -> Discrete Varying Lowpass/1
  Constant/1 -> Discrete Varying Lowpass/2
  Saturation2/1 -> Yaw/1
  In3/1 -> Multiply2/1

== system RL_SAC/Attitude Control/Subsystem3 ==
  In1 : Inport
  In2 : Inport  Port=2
  In3 : Inport  Port=3
  Add : Sum  Inputs=++-
  Constant : Constant  Value=5
  Discrete Varying Lowpass : cstblocks/Linear Parameter Varying/Discrete Varying Lowpass  N=1  w0=0  Ts=1e-2
  Discrete-Time Integrator : DiscreteIntegrator  SampleTime=-1  ICPrevOutput=DiscIntNeverNeededParam  ICPrevScaledInput=DiscIntNeverNeededParam
  Multiply1 : Gain  Gain=0.3
  Multiply2 : Gain  Gain=0.01
  Multiply3 : Gain  Gain=0
  Multiply4 : Gain
  Saturation2 : Saturate  UpperLimit=20  LowerLimit=-20
  Sum3 : Sum  Inputs=|+-
  Roll : Outport
  wires:
  In1/1 -> Sum3/1
  Sum3/1 -> Multiply1/1
  In2/1 -> Sum3/2
  Discrete-Time Integrator/1 -> Multiply3/1
  Multiply3/1 -> Add/2
  Discrete Varying Lowpass/1 -> Multiply4/1
  Multiply1/1 -> Add/1, Discrete-Time Integrator/1
  Multiply4/1 -> Add/3
  Add/1 -> Saturation2/1
  Multiply2/1 -> Discrete Varying Lowpass/1
  Constant/1 -> Discrete Varying Lowpass/2
  Saturation2/1 -> Roll/1
  In3/1 -> Multiply2/1

== system RL_SAC/Attitude Control/Subsystem4 ==
  In1 : Inport
  In2 : Inport  Port=2
  In3 : Inport  Port=3
  Add : Sum  Inputs=++-
  Constant : Constant  Value=5
  Discrete Varying Lowpass : cstblocks/Linear Parameter Varying/Discrete Varying Lowpass  N=1  w0=0  Ts=1e-2
  Discrete-Time Integrator : DiscreteIntegrator  SampleTime=-1  ICPrevOutput=DiscIntNeverNeededParam  ICPrevScaledInput=DiscIntNeverNeededParam
  Multiply1 : Gain  Gain=0.3
  Multiply2 : Gain  Gain=0.01
  Multiply3 : Gain  Gain=0
  Multiply4 : Gain
  Saturation2 : Saturate  UpperLimit=20  LowerLimit=-20
  Sum3 : Sum  Inputs=|+-
  Pitch : Outport
  wires:
  In1/1 -> Sum3/1
  Sum3/1 -> Multiply1/1
  In2/1 -> Sum3/2
  Discrete-Time Integrator/1 -> Multiply3/1
  Multiply3/1 -> Add/2
  Discrete Varying Lowpass/1 -> Multiply4/1
  Multiply1/1 -> Add/1, Discrete-Time Integrator/1
  Multiply4/1 -> Add/3
  Add/1 -> Saturation2/1
  Multiply2/1 -> Discrete Varying Lowpass/1
  Constant/1 -> Discrete Varying Lowpass/2
  Saturation2/1 -> Pitch/1
  In3/1 -> Multiply2/1

== system RL_SAC/Attitude Control/Subsystem5 ==
  "  " : Inport
  Selector : Selector  InputPortWidth=3  IndexOptions=Index vector (dialog)  Indices=[1]  OutputSizes=1
  Selector1 : Selector  InputPortWidth=3  IndexOptions=Index vector (dialog)  Indices=[2]  OutputSizes=1
  Selector2 : Selector  InputPortWidth=3  IndexOptions=Index vector (dialog)  Indices=[3]  OutputSizes=1
  Out1 : Outport
  Out2 : Outport  Port=2
  Out3 : Outport  Port=3
  wires:
  Selector2/1 -> Out3/1
  Selector1/1 -> Out2/1
  Selector/1 -> Out1/1
  "  "/1 -> Selector2/1, Selector/1, Selector1/1

== system RL_SAC/Attitude Control/Subsystem6 ==
  "  " : Inport
  Selector : Selector  InputPortWidth=3  IndexOptions=Index vector (dialog)  Indices=[1]  OutputSizes=1
  Selector1 : Selector  InputPortWidth=3  IndexOptions=Index vector (dialog)  Indices=[2]  OutputSizes=1
  Selector2 : Selector  InputPortWidth=3  IndexOptions=Index vector (dialog)  Indices=[3]  OutputSizes=1
  Out1 : Outport
  Out2 : Outport  Port=2
  Out3 : Outport  Port=3
  wires:
  "  "/1 -> Selector1/1, Selector/1, Selector2/1
  Selector/1 -> Out1/1
  Selector1/1 -> Out2/1
  Selector2/1 -> Out3/1

== system RL_SAC/Gyro/noise ==
  In1 : Inport
  Add1 : Sum
  Add2 : Sum
  Add3 : Sum
  Band-Limited White Noise : simulink/Sources/Band-Limited White Noise  Cov=[1e-6]  Ts=1e-2  seed=[23341]
  Band-Limited White Noise1 : simulink/Sources/Band-Limited White Noise  Cov=[1e-6]  Ts=1e-2  seed=[23345]
  Band-Limited White Noise2 : simulink/Sources/Band-Limited White Noise  Cov=[1e-6]  Ts=1e-2  seed=[22341]
  Mux : Mux  Inputs=3
  Subsystem1 : Subsystem
  Out1 : Outport
  wires:
  In1/1 -> Subsystem1/1("  ")
  Mux/1 -> Out1/1
  Band-Limited White Noise/1 -> Add1/2
  Band-Limited White Noise1/1 -> Add2/2
  Band-Limited White Noise2/1 -> Add3/2
  Subsystem1/1(Out1) -> Add1/1
  Subsystem1/2(Out2) -> Add2/1
  Subsystem1/3(Out3) -> Add3/1
  Add1/1 -> Mux/1
  Add2/1 -> Mux/2
  Add3/1 -> Mux/3

== system RL_SAC/Linear State Estimator/Complimentary filter ==
  In1 : Inport
  f_lin_pos : Inport  Port=2
  Constant : Constant  Value=2
  Discrete Transfer Fcn : DiscreteTransferFcn  Numerator=[4]  Denominator=[4 1]
  Discrete Varying Lowpass : cstblocks/Linear Parameter Varying/Discrete Varying Lowpass  N=1  w0=0  Ts=1e-2
  Sum : Sum  Inputs=|++
  F_Lin_Pos : Outport
  wires:
  Constant/1 -> Discrete Varying Lowpass/2
  In1/1 -> Discrete Transfer Fcn/1
  Discrete Varying Lowpass/1 -> Sum/1
  Discrete Transfer Fcn/1 -> Sum/2
  f_lin_pos/1 -> Discrete Varying Lowpass/1
  Sum/1 -> F_Lin_Pos/1

== system RL_SAC/Position Control/Subsystem ==
  In1 : Inport
  In2 : Inport  Port=2
  Add : Sum  Inputs=++-
  Constant : Constant  Value=5
  Discrete Derivative : simulink/Discrete/Discrete Derivative  gainval=1.0  ICPrevScaledInput=0.0  OutMin=[]  OutMax=[]  OutDataType=fixdt(1, 16)  OutScaling=2^-10  DoSatur=off
  Discrete Varying Lowpass : cstblocks/Linear Parameter Varying/Discrete Varying Lowpass  N=1  w0=0  Ts=1e-2
  Discrete-Time Integrator : DiscreteIntegrator  SampleTime=-1  ICPrevOutput=DiscIntNeverNeededParam  ICPrevScaledInput=DiscIntNeverNeededParam
  Multiply1 : Gain  Gain=0.15
  Multiply2 : Gain  Gain=0.3
  Multiply3 : Gain  Gain=12
  Sum : Sum  Inputs=|+-
  Des Thrust : Outport
  wires:
  In1/1 -> Sum/1
  Discrete Varying Lowpass/1 -> Discrete Derivative/1
  Discrete Derivative/1 -> Multiply2/1
  Discrete-Time Integrator/1 -> Multiply1/1
  Sum/1 -> Multiply3/1
  Multiply3/1 -> Add/1, Discrete-Time Integrator/1
  Multiply1/1 -> Add/2
  Multiply2/1 -> Add/3
  Add/1 -> Des Thrust/1
  Constant/1 -> Discrete Varying Lowpass/2
  In2/1 -> Sum/2, Discrete Varying Lowpass/1

== system RL_SAC/Position Control/Subsystem1 ==
  "  " : Inport
  Selector : Selector  InputPortWidth=3  IndexOptions=Index vector (dialog)  Indices=[1]  OutputSizes=1
  Selector1 : Selector  InputPortWidth=3  IndexOptions=Index vector (dialog)  Indices=[2]  OutputSizes=1
  Selector2 : Selector  InputPortWidth=3  IndexOptions=Index vector (dialog)  Indices=[3]  OutputSizes=1
  Out1 : Outport
  Out2 : Outport  Port=2
  Out3 : Outport  Port=3
  wires:
  Selector2/1 -> Out3/1
  Selector1/1 -> Out2/1
  Selector/1 -> Out1/1
  "  "/1 -> Selector2/1, Selector/1, Selector1/1

== system RL_SAC/Position Control/Subsystem2 ==
  "  " : Inport
  Selector : Selector  InputPortWidth=3  IndexOptions=Index vector (dialog)  Indices=[1]  OutputSizes=1
  Selector1 : Selector  InputPortWidth=3  IndexOptions=Index vector (dialog)  Indices=[2]  OutputSizes=1
  Selector2 : Selector  InputPortWidth=3  IndexOptions=Index vector (dialog)  Indices=[3]  OutputSizes=1
  Out2 : Outport
  Out1 : Outport  Port=2
  Out3 : Outport  Port=3
  wires:
  Selector2/1 -> Out3/1
  "  "/1 -> Selector2/1, Selector/1, Selector1/1
  Selector1/1 -> Out1/1
  Selector/1 -> Out2/1

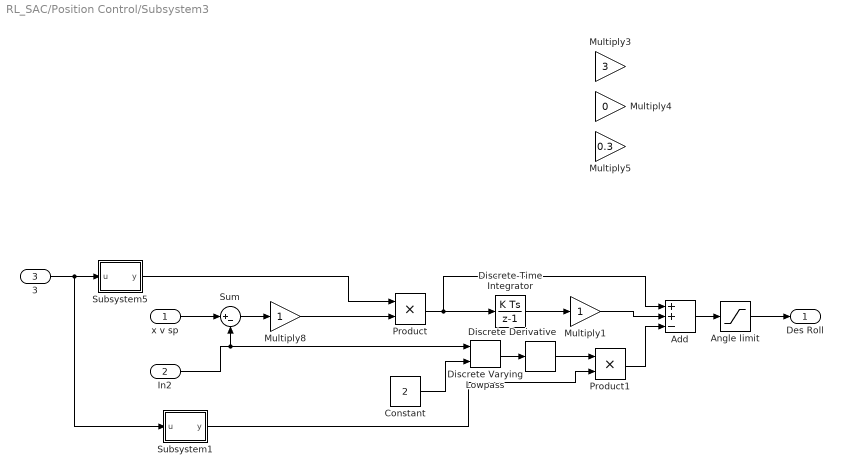
== system RL_SAC/Position Control/Subsystem3 ==
  x v sp : Inport
  In2 : Inport  Port=2
  3 : Inport  Port=3
  Add : Sum  Inputs=++-
  Angle limit : Saturate  UpperLimit=0.785  LowerLimit=-0.785
  Constant : Constant  Value=2
  Discrete Derivative : simulink/Discrete/Discrete Derivative  gainval=1.0  ICPrevScaledInput=0.0  OutMin=[]  OutMax=[]  OutDataType=fixdt(1, 16)  OutScaling=2^-10  DoSatur=off
  Discrete Varying Lowpass : cstblocks/Linear Parameter Varying/Discrete Varying Lowpass  N=1  w0=0  Ts=1e-2
  Discrete-Time Integrator : DiscreteIntegrator  SampleTime=-1  ICPrevOutput=DiscIntNeverNeededParam  ICPrevScaledInput=DiscIntNeverNeededParam
  Multiply1 : Gain
  Multiply3 : Gain  Gain=3
  Multiply4 : Gain  Gain=0
  Multiply5 : Gain  Gain=0.3
  Multiply8 : Gain
  Product : Product
  Product1 : Product
  Subsystem1 : Subsystem
  Subsystem5 : Subsystem
  Sum : Sum  Inputs=|+-
  Des Roll : Outport
  wires:
  Add/1 -> Angle limit/1
  Multiply1/1 -> Add/2
  Sum/1 -> Multiply8/1
  Discrete-Time Integrator/1 -> Multiply1/1
  Discrete Derivative/1 -> Product1/1
  Discrete Varying Lowpass/1 -> Discrete Derivative/1
  Product/1 -> Add/1, Discrete-Time Integrator/1
  Product1/1 -> Add/3
  3/1 -> Subsystem5/1(u), Subsystem1/1(u)
  In2/1 -> Discrete Varying Lowpass/1, Sum/2
  x v sp/1 -> Sum/1
  Multiply8/1 -> Product/2
  Angle limit/1 -> Des Roll/1
  Constant/1 -> Discrete Varying Lowpass/2
  Subsystem5/1(y) -> Product/1
  Subsystem1/1(y) -> Product1/2

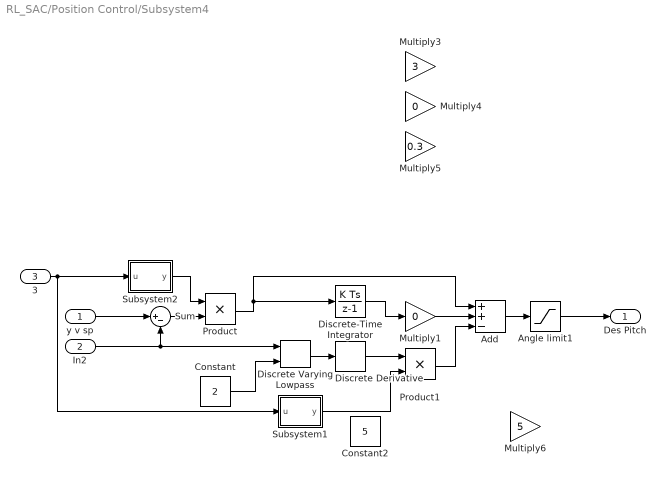
== system RL_SAC/Position Control/Subsystem4 ==
  y v sp : Inport
  In2 : Inport  Port=2
  3 : Inport  Port=3
  Add : Sum  Inputs=++-
  Angle limit1 : Saturate  UpperLimit=0.785  LowerLimit=-0.785
  Constant : Constant  Value=2
  Constant2 : Constant  Value=5
  Discrete Derivative : simulink/Discrete/Discrete Derivative  gainval=1.0  ICPrevScaledInput=0.0  OutMin=[]  OutMax=[]  OutDataType=fixdt(1, 16)  OutScaling=2^-10  DoSatur=off
  Discrete Varying Lowpass : cstblocks/Linear Parameter Varying/Discrete Varying Lowpass  N=1  w0=0  Ts=1e-2
  Discrete-Time Integrator : DiscreteIntegrator  SampleTime=-1  ICPrevOutput=DiscIntNeverNeededParam  ICPrevScaledInput=DiscIntNeverNeededParam
  Multiply1 : Gain  Gain=0
  Multiply3 : Gain  Gain=3
  Multiply4 : Gain  Gain=0
  Multiply5 : Gain  Gain=0.3
  Multiply6 : Gain  Gain=5
  Product : Product
  Product1 : Product
  Subsystem1 : Subsystem
  Subsystem2 : Subsystem
  Sum : Sum  Inputs=|+-
  Des Pitch : Outport
  wires:
  Subsystem1/1(y) -> Product1/2
  Product1/1 -> Add/3
  Subsystem2/1(y) -> Product/1
  3/1 -> Subsystem1/1(u), Subsystem2/1(u)
  Product/1 -> Add/1, Discrete-Time Integrator/1
  In2/1 -> Discrete Varying Lowpass/1, Sum/2
  Angle limit1/1 -> Des Pitch/1
  y v sp/1 -> Sum/1
  Discrete Varying Lowpass/1 -> Discrete Derivative/1
  Discrete Derivative/1 -> Product1/1
  Discrete-Time Integrator/1 -> Multiply1/1
  Sum/1 -> Product/2
  Multiply1/1 -> Add/2
  Add/1 -> Angle limit1/1
  Constant/1 -> Discrete Varying Lowpass/2

== system RL_SAC/Position Control/Subsystem5 ==
  u : Inport
  Abs1 : Abs  SaturateOnIntegerOverflow=off
  MATLAB Function : MATLAB Function  TreatAsAtomicUnit=on
  y : Outport
  wires:
  MATLAB Function/1(y) -> y/1
  u/1 -> Abs1/1
  Abs1/1 -> MATLAB Function/1(u)

== system RL_SAC/Position Control/Subsystem6 ==
  u : Inport
  Abs1 : Abs  SaturateOnIntegerOverflow=off
  MATLAB Function : MATLAB Function  TreatAsAtomicUnit=on
  y : Outport
  wires:
  MATLAB Function/1(y) -> y/1
  u/1 -> Abs1/1
  Abs1/1 -> MATLAB Function/1(u)
